simulink model "motorusingnn"  (R2017b)
settings: Solver=VariableStepAuto  StartTime=0.0  StopTime=10.0  RelTol=1e-3
undefined symbols (not defined in the file or in its folder): sigbuilder_block
libraries: neural x1, simulink x1
settings Model: Creator=AMAN  LastModifiedBy=AMAN

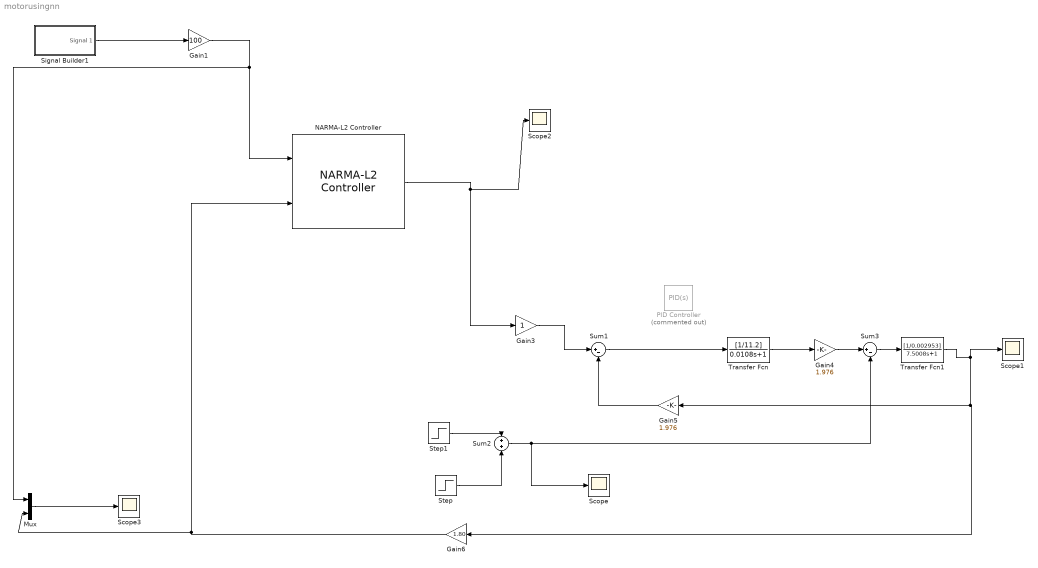
== system motorusingnn ==
  Gain1 : Gain  Gain=100
  Gain3 : Gain
  Gain4 : Gain  Gain=1.976
  Gain5 : Gain  Gain=1.976
  Gain6 : Gain  Gain=1.80
  Mux : Mux  Inputs=2
  NARMA-L2 Controller : neural/Control Systems/NARMA-L2 Controller  Normalize=1  IW1_1=[-0.89287723045770839292 1.3725849506216476481 0.93956657401429055643;2.4567282064623419124 -2.2642702901876381461 -2.0402569116097910573;-5.5846656182079890129 2.4880452703757693911 1.9125922405741966337;-2.3346263152111643713 1.264811725532398734 0.79431304010182324227;1.1537358138881068648 0.97712828817821140159 -1.0312317079078880955;1.9532300853608552949 -0.12097647363935662423 1.0606044393284863592;-3.2851334176565569756 1.3064519086479284837 0.12475023271769368483]  IW3_2=[2.2142443107492764121 2.7679175507303113157 -0.75015211591374830746;4.2263022697693068963 -2.0935820550035635357 -1.5319929846568289822;3.0970909910080073324 0.96481527060338945212 -0.8213601722874468436;-0.61238330404696061926 -2.2444551029508876816 -0.82299823907081282037;-1.561028782633493428 -1.2580929976168624407 2.3119120057146029801;-0.16135118034053252956 0.72763127440677277669 0.41854296252098177611;1.9150668300171138636 -1.5039512915434258833 0.30287764045543291713]  IW5_3=-0.42360049198449944985  LW2_1=[-1.4208534634428151566 -0.53576982480740054093 0.50431439138105338404 -1.2455073424626477152 -0.011307218692920671319 -0.37644988523150541004 -1.7653822498394506901]  LW4_3=[0.10247451397453792576 3.327161140972704878 0.51384889094017982547 0.35243995582624276786 0.729377149561631688 -1.3033949193537894828 -1.8316557318053152681]  LW5_4=-0.370761473743167147  LW6_5=-0.36281687348923574721  LW6_2=-1.6833929762691062226  B1=[3.0166258810940766999;-2.6529254864613402987;0.55059501115687137229;0.68120908546479508328;1.5462349466943117182;2.4842678160881059846;-2.6952325425993493013]  B2=-0.013505602475753065647  B3=[-1.4654464022461186623;-1.4236043017339581329;0.59630558727058946555;-0.49150425134488717749;-1.1266793987621301909;3.5362641176005729093;3.1429803010435644062]  B4=-1.8893241277228471908  Limit_output=0  min_output=-Inf  max_output=Inf  Use_Previous_Weights=1  Ts=0.03  S1=7  Ni=3  Nj=1  sim_file=motorref  trainfun=trainlm  Use_validation=0  Use_Testing=1  max_i=240  min_i=0  max_i_int=40  min_i_int=0.0001  sam_training=500  epochs=150  minp=30.47683591044145146  maxp=229.80164050423141475  mint=0  maxt=229.80164050423141475
      settings: SourceProductName=Neural Network Toolbox  SourceProductBaseCode=NN
  PID Controller : simulink/Continuous/PID Controller  Commented=on  Controller=PID  TimeDomain=Continuous-time  SampleTime=-1  IntegratorMethod=Forward Euler  FilterMethod=Forward Euler  Form=Parallel  UseFilter=on  ControllerParametersSource=internal  P=1  I=1  D=0  N=100  InitialConditionSource=internal  InitialConditionForIntegrator=0  InitialConditionForFilter=0  ExternalReset=none  LimitOutput=off  UpperSaturationLimit=inf  LowerSaturationLimit=-inf  LinearizeAsGain=on  AntiWindupMode=none  Kb=1  TrackingMode=off  Kt=1  PParamMin=[]  PParamMax=[]  IParamMin=[]  IParamMax=[]  DParamMin=[]  DParamMax=[]  NParamMin=[]  NParamMax=[]  KbParamMin=[]  KbParamMax=[]  KtParamMin=[]  KtParamMax=[]  POutMin=[]  POutMax=[]  IOutMin=[]  IOutMax=[]  DOutMin=[]  DOutMax=[]  NOutMin=[]  NOutMax=[]  KbOutMin=[]  KbOutMax=[]  KtOutMin=[]  KtOutMax=[]  IntegratorOutMin=[]  IntegratorOutMax=[]  FilterOutMin=[]  FilterOutMax=[]  SumOutMin=[]  SumOutMax=[]  SumI1OutMin=[]  SumI1OutMax=[]  SumI2OutMin=[]  SumI2OutMax=[]  SumI3OutMin=[]  SumI3OutMax=[]  SumDOutMin=[]  SumDOutMax=[]  SaturationOutMin=[]  SaturationOutMax=[]  IntegratorContinuousStateAttributes=''  IntegratorStateMustResolveToSignalObject=off  IntegratorRTWStateStorageClass=Auto  FilterContinuousStateAttributes=''  FilterStateMustResolveToSignalObject=off  FilterRTWStateStorageClass=Auto  DifferentiatorICPrevScaledInput=0  DifferentiatorOutMin=[]  DifferentiatorOutMax=[]  InitialConditionSetting=State (most efficient)  FilterDiffOutCoefMin=[]  FilterDiffOutCoefMax=[]  SumDenOutMin=[]  SumDenOutMax=[]  SumNumOutMin=[]  SumNumOutMax=[]  ReciprocalOutMin=[]  ReciprocalOutMax=[]  DivideOutMin=[]  DivideOutMax=[]  TunerSelectOption=Transfer Function Based (PID Tuner App)
  Scope{,1..3} (4 alike) : Scope
  Signal Builder1 : Subsystem  Tag=STV Subsys  LoadFcn=sigbuilder_block('load');  StartFcn=sigbuilder_block('start');  StopFcn=sigbuilder_block('stop');  ClipboardFcn=sigbuilder_block('clipboard');  mask(Sigbuilder block){tuvar=[0:10]}
      mask help: Simulink:masks:SigbuilderBlock_MD
      mask init:
      | if ~strcmp(get_param(bdroot(gcbh),'SimulationStatus'),'stopped') tuvar = sigbuilder_block('maskInit'); end
      settings: CopyFcn=sigbuilder_block('copy');  DeleteFcn=sigbuilder_block('delete');  ModelCloseFcn=sigbuilder_block('modelClose');  PreSaveFcn=sigbuilder_block('preSave');  PauseFcn=sigbuilder_block('pause');  ContinueFcn=sigbuilder_block('continue');  NameChangeFcn=sigbuilder_block('namechange');  OpenFcn=sigbuilder_block('open',[437.6 199.2 550.4 400 ]);  CloseFcn=sigbuilder_block('close');
      mask Display: plot(0, 0, 100, 100,[2, 2, 32, 32, 2], [68, 8, 8, 68, 68],[32, 2], [38, 38], [32, 19, 2],[53, 60, 44], [32, 17, 17, 2],[16, 16, 31, 31]);txt = getActiveGroup(gcbh);text(2, 100, txt,'verticalAlignment', 'top');
  Step : Step  After=0.5  SampleTime=0
  Step1 : Step  Time=0  After=0.2  SampleTime=0
  Sum1 : Sum  Inputs=|+-
  Sum2 : Sum
  Sum3 : Sum  Inputs=|+-
  Transfer Fcn : TransferFcn  Numerator=[1/11.2]  Denominator=[0.0108 1]
  Transfer Fcn1 : TransferFcn  Numerator=[1/0.002953]  Denominator=|
      | [7.5008
      |  1]
  wires:
  Gain5/1 -> Sum1/2
  Mux/1 -> Scope3/1
  Gain6/1 -> Mux/2, NARMA-L2 Controller/2
  Gain3/1 -> Sum1/1
  NARMA-L2 Controller/1 -> Scope2/1, Gain3/1
  Gain4/1 -> Sum3/1
  Transfer Fcn1/1 -> Gain5/1, Gain6/1, Scope1/1
  Step1/1 -> Sum2/1
  Transfer Fcn/1 -> Gain4/1
  Sum2/1 -> Scope/1, Sum3/2
  Sum1/1 -> Transfer Fcn/1
  Sum3/1 -> Transfer Fcn1/1
  Step/1 -> Sum2/2
  Gain1/1 -> Mux/1, NARMA-L2 Controller/1
  Signal Builder1/1(Signal 1) -> Gain1/1

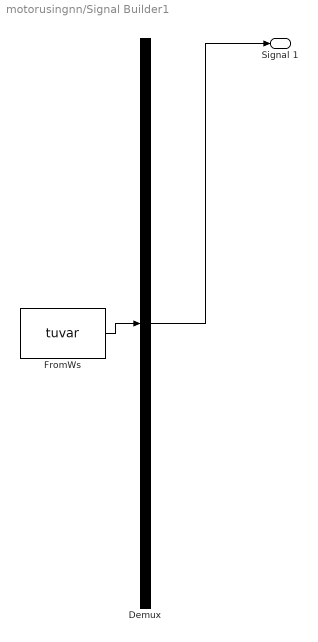
== system motorusingnn/Signal Builder1 ==
  Demux : Demux  Tag=STV Demux  Outputs=1
  FromWs : FromWorkspace  Tag=STV FromWs  VariableName=tuvar  SampleTime=0
      SigBuilderData=|
      | common.afterFinalStr = 'Extrapolate'
      | common.sampleTime = 0
      | dataSet.timeRange = [0 10]
      | dataSet.name = 'Group 1'
      | sbobj.Groups.Name = 'Group 1'
      | sbobj.Groups.Signals.Name = 'Signal 1'
      | sbobj.Groups.Signals.XData = [0 4 4 6 6 10]
      | sbobj.Groups.Signals.YData = [0.78 0.82 1 1 0.585 -0.07]
  Signal 1 : Outport  Tag=STV Outport
  wires:
  Demux/1 -> Signal 1/1
  FromWs/1 -> Demux/1
